simulink model "ProjectOfPreCrashSafetySystem"  (R2016b)
settings: Solver=VariableStepAuto  StartTime=0.0  StopTime=10.0  RelTol=1e-3
settings Model: Creator=Takiya  LastModifiedBy=Takiya

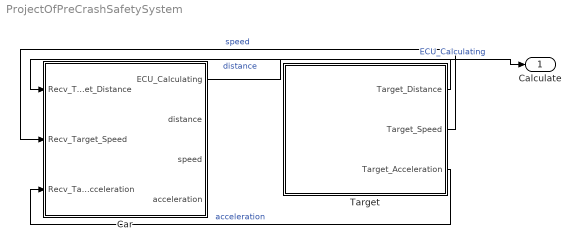
== system ProjectOfPreCrashSafetySystem ==
  Car : Subsystem
  Target : Subsystem
      settings: AttributesFormatString=TargetCar
  Calculate : Outport
      settings: AttributesFormatString=ECU_Calculating
  wires:
  Target/3(Target_Acceleration) -> Car/3(Recv_Target_Acceleration)  "acceleration"
  Target/1(Target_Distance) -> Car/1(Recv_Target_Distance)  "distance"
  Target/2(Target_Speed) -> Car/2(Recv_Target_Speed)  "speed"
  Car/1(ECU_Calculating) -> Calculate/1  "ECU_Calculating"

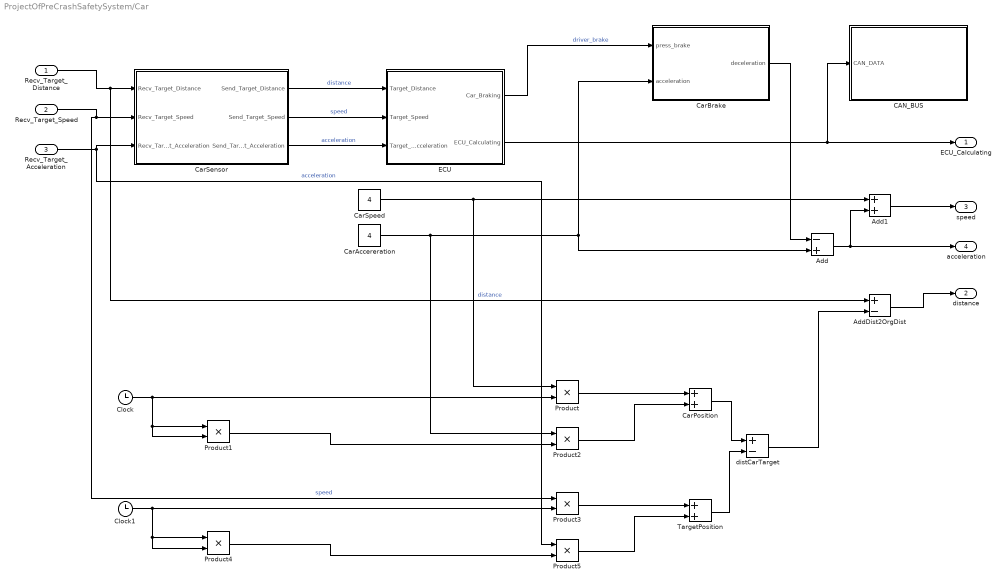
== system ProjectOfPreCrashSafetySystem/Car ==
  Recv_Target_Distance : Inport
      settings: AttributesFormatString=distance
  Recv_Target_Speed : Inport  Port=2
      settings: AttributesFormatString=speed
  Recv_Target_Acceleration : Inport  Port=3
      settings: AttributesFormatString=acceleration
  Add : Sum  Inputs=-+
  Add1 : Sum
  AddDist2OrgDist : Sum  Inputs=+-
  CAN_BUS : Subsystem
  CarAccereration : Constant  Value=4
  CarBrake : Subsystem
      settings: AttributesFormatString=Brake
  CarPosition : Sum
  CarSensor : Subsystem
      settings: AttributesFormatString=Sensor
  CarSpeed : Constant  Value=4
  Clock : Clock
  Clock1 : Clock
  ECU : Subsystem
  Product{,1..5} (6 alike) : Product
  TargetPosition : Sum
  distCarTarget : Sum  Inputs=+-
  ECU_Calculating : Outport
  distance : Outport  Port=2
  speed : Outport  Port=3
  acceleration : Outport  Port=4
  wires:
  CarSensor/3(Send_Target_Acceleration) -> ECU/3(Target_Acceleration)  "acceleration"
  CarSensor/1(Send_Target_Distance) -> ECU/1(Target_Distance)  "distance"
  CarSensor/2(Send_Target_Speed) -> ECU/2(Target_Speed)  "speed"
  ECU/1(Car_Braking) -> CarBrake/1(press_brake)  "driver_brake"
  ECU/2(ECU_Calculating) -> CAN_BUS/1(CAN_DATA), ECU_Calculating/1
  Recv_Target_Distance/1 -> CarSensor/1(Recv_Target_Distance), AddDist2OrgDist/1  "distance"
  Recv_Target_Speed/1 -> Product3/1, CarSensor/2(Recv_Target_Speed)  "speed"
  Recv_Target_Acceleration/1 -> Product5/1, CarSensor/3(Recv_Target_Acceleration)  "acceleration"
  CarAccereration/1 -> Product2/1, CarBrake/2(acceleration), Add/2
  CarBrake/1(deceleration) -> Add/1
  Add/1 -> Add1/2, acceleration/1
  CarSpeed/1 -> Product/1, Add1/1
  Add1/1 -> speed/1
  Clock/1 -> Product1/2, Product1/1, Product/2
  Product1/1 -> Product2/2
  Product2/1 -> CarPosition/2
  Product/1 -> CarPosition/1
  Clock1/1 -> Product3/2, Product4/1, Product4/2
  Product4/1 -> Product5/2
  Product5/1 -> TargetPosition/2
  Product3/1 -> TargetPosition/1
  CarPosition/1 -> distCarTarget/1
  TargetPosition/1 -> distCarTarget/2
  distCarTarget/1 -> AddDist2OrgDist/2
  AddDist2OrgDist/1 -> distance/1

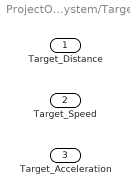
== system ProjectOfPreCrashSafetySystem/Target ==
  Target_Distance : Outport
      settings: AttributesFormatString=distance
  Target_Speed : Outport  Port=2
      settings: AttributesFormatString=speed
  Target_Acceleration : Outport  Port=3
      settings: AttributesFormatString=acceleration

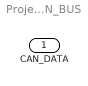
== system ProjectOfPreCrashSafetySystem/Car/CAN_BUS ==
  CAN_DATA : Inport
      settings: AttributesFormatString=ECU_Calculating

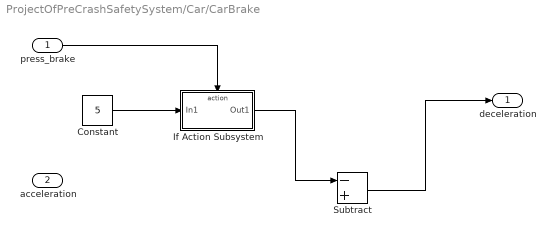
== system ProjectOfPreCrashSafetySystem/Car/CarBrake ==
  press_brake : Inport
      settings: AttributesFormatString=driver_brake
  acceleration : Inport  Port=2
  Constant : Constant  Value=5
  If Action Subsystem : Subsystem  TreatAsAtomicUnit=on
  Subtract : Sum  Inputs=-+
  deceleration : Outport
      settings: AttributesFormatString=acceleration
  wires:
  press_brake/1 -> If Action Subsystem/Action
  Subtract/1 -> deceleration/1
  If Action Subsystem/1(Out1) -> Subtract/1
  Constant/1 -> If Action Subsystem/1(In1)

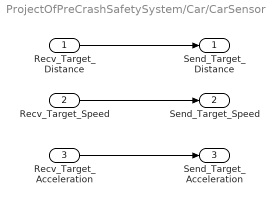
== system ProjectOfPreCrashSafetySystem/Car/CarSensor ==
  Recv_Target_Distance : Inport
      settings: AttributesFormatString=distance
  Recv_Target_Speed : Inport  Port=2
      settings: AttributesFormatString=speed
  Recv_Target_Acceleration : Inport  Port=3
      settings: AttributesFormatString=acceleration
  Send_Target_Distance : Outport
      settings: AttributesFormatString=distance
  Send_Target_Speed : Outport  Port=2
      settings: AttributesFormatString=speed
  Send_Target_Acceleration : Outport  Port=3
      settings: AttributesFormatString=acceleration
  wires:
  Recv_Target_Distance/1 -> Send_Target_Distance/1
  Recv_Target_Speed/1 -> Send_Target_Speed/1
  Recv_Target_Acceleration/1 -> Send_Target_Acceleration/1

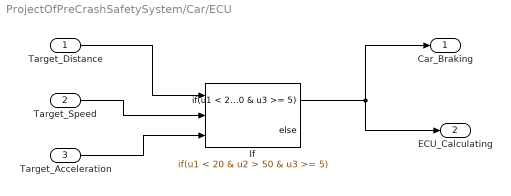
== system ProjectOfPreCrashSafetySystem/Car/ECU ==
  Target_Distance : Inport
      settings: AttributesFormatString=distance
  Target_Speed : Inport  Port=2
      settings: AttributesFormatString=speed
  Target_Acceleration : Inport  Port=3
      settings: AttributesFormatString=acceleration
  If : If  NumInputs=3  IfExpression=u1 < 20 & u2 > 50 & u3 >= 5
  Car_Braking : Outport
      settings: AttributesFormatString=driver_brake
  ECU_Calculating : Outport  Port=2
  wires:
  Target_Distance/1 -> If/1
  Target_Speed/1 -> If/2
  Target_Acceleration/1 -> If/3
  If/1 -> ECU_Calculating/1, Car_Braking/1

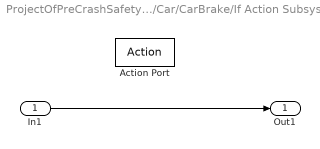
== system ProjectOfPreCrashSafetySystem/Car/CarBrake/If Action Subsystem ==
  In1 : Inport
  Action Port : ActionPort
  Out1 : Outport
  wires:
  In1/1 -> Out1/1
